simulink model "trans_canal_recep_2015a"  (R2015a)
settings: Solver=ode45  SolverMode=SingleTasking  StartTime=0.0  StopTime=100  MaxStep=0.001  RelTol=1e-3
InitFcn:
  | cd(tempdir)
  | clearvars
  | clc
  | 
  | %Carrossel?
  | mode_t=1;
  | 
  | %Depuração?
  | dep=0;
  | 
  | %Parâmetros do transmissor
  | fs_Tx=200e3;
  | f_bits=10e3;
  | rolloff=0.5;
  | smpl_per_symb=5;
  | [N,D]=rat(400000/(f_bits*smpl_per_symb));
  | rate_inter=(N);
  | rate_dec=(D);
  | 
  | %Canal
  | noise_pwr=0.25;
  | freq_canal=500;
  | att_canal=0.001;
  | 
  | 
  | %Barker e coef. do filtro casado
  | bark=[3 3 3 3 3 0 0 3 3 0 3 0 3 3 3 2 1 2 2 3 3 3 0 3 1 1];
  | y = pskmod(bark,4,pi/4,'gray');
  | coef=flip(conj(y));
  | 
  | 
  | %%%RECEPTOR%%%
  | 
  | Rsymbol = f_bits/2;                     % QPSK, so 2 samples per symbol
  | fs_Rx = 240e3;                            % sampling rate in the receiver
  | Rx_dec=6;
  | Rx_int=2;
  | OSR = (fs_Rx*Rx_int/(Rx_dec))/Rsymbol;     % oversampling ratio used in timing and frequency synch
  | smpl_per_symb_rec=fs_Rx/(Rx_dec*Rsymbol);
  | 
  | if f_bits==2e3
  |    nbw=0.00095;
  |    zeta=1.2;
  | else
  |    nbw=0.001;
  |    zeta=1.1;
  | end
  | 
  | %Largura de banda norm. do sinc. de portadora
  | if f_bits==40e3
  |     c_nbw=0.05;
  | else
  |     c_nbw=0.1;
  | end
  | 
  | %data='The man in black fled across the desert, and the gunslinger followed. The desert was the apotheosis of all deserts, huge, standing to the sky for what might have been parsecs in all directions. White; blinding; waterless; without feature save for the faint, cloudy haze of the mountains which sketched themselves on the horizon and the devil-grass which brought sweet dreams, nightmares, death. An occasional tombstone sign pointed the way, for once the drifted track that cut its way through the thick crust of alkali had been a highway and coaches had followed it. The world had moved on since then. The world had emptied. The gunslinger walked stolidly, not hurrying, not loafing. A hide waterbag was slung around his middle like a bloated sausage. It was almost full. He had progressed through the khef over many years, and had reached the fifth level. At the seventh or eighth, he would not have been thirsty; he could have watched own body dehydrate with clinical, detached attention, watering its crevices and dark inner hollows only when his logic told him it must be done. He was not seventh or eighth. He was fifth. So he was thirsty, although he had no particular urge to drink. In a vague way, all this pleased him. It was romantic. Below the waterbag were his guns, finely weighted to his hand. The two belts crisscrossed above his crotch. The holsters were oiled too deeply for even this Philistine sun to crack. The stocks of the guns were sandalwood, yellow and finely grained. The holsters were tied down with raw hide cord, and they swung heavily against his hips. The brass casings of the cartridges looped into the gun belts twinkled and flashed and heliographed in the sun. The leather made subtle creaking noises. The guns themselves made no noise. They had spilled blood. There was no need to make noise in the sterility of the desert His clothes were the no-color of rain or dust. His shirt was open at the throat, with a rawhide thong dangling loosely in hand-punched eyelets. His pants were seam-stretched dungarees. He breasted a gently rising dune (although there was no sand here; the desert was hardpan, and even the harsh winds that blew when dark came raised only an aggravating harsh dust like scouring powder) and saw the kicked remains of a tiny campfire on the lee side, the side which the sun would quit earliest. Small signs like this, once more affirming the man in black´s essential humanity, never failed to please him. His lips stretched in the pitted, flaked remains of his face. He squatted. He had burned the devil-grass, of course. It was the only thing out here that would burn. It burned with a greasy, flat light, and it burned slow. Border dwellers had told him that devils lived even in the flames. They burned it but would not look into the light. They said the devils hypnotized, beckoned, would eventually draw the one who looked into the fires. And the next man foolish enough to look into the fire might see you. The burned grass was crisscrossed in the now-familiar ideographic pattern, and crumbled to gray senselessness before the gunslinger´s prodding hand. There was nothing in the remains but a charred scrap of bacon, which he ate thoughtfully. It had always been this way. The gunslinger had followed the man in black across the desert for two months now, across the endless, screamingly monotonous purgatorial wastes, and had yet to find spoor other than the hygienic sterile ideographs of the man in black´s camp fires. He had not found a can, a bottle, or a waterbag (the gunslinger had left four of those behind, like dead snake-skins).';
  | data='The man in black fled across the desert, and the gunslinger followed. The desert was the apotheosis of all deserts, huge, standing to the sky for what might have been parsecs in all directions. White; blinding; waterless; without feature save for the faint, cloudy haze of the mountains which sketched themselves on the horizon and the devil-grass which brought sweet dreams, nightmares, death. An occasional tombstone sign pointed the way, for once the drifted track that cut its way through the thick crust of alkali had been a highway and coaches had followed it. The world had moved on since then.';
undefined symbols (not defined in the file): firnyquist, jsin
libraries: dspmlti4 x5, commdigbbndpm3 x3, dspsrcs4 x2, commfilt2 x2, commrfcorlib x1, simulink x1
settings Model: CovMetricSettings=dwe  CovHtmlReporting=off  covSaveCumulativeToWorkspaceVar=off  CovSaveSingleToWorkspaceVar=off  CovExternalEMLEnable=on  Creator=Enrique Pinto  LastModifiedBy=Enrique Pinto
settings DataIOCC: LimitDataPoints=off  SaveFormat=Dataset
settings DebuggingCC: SFUnexpectedBacktrackingDiag=error  SFNoUnconditionalDefaultTransitionDiag=error
settings HardwareCC: ProdBitPerPointer=64  ProdLargestAtomicFloat=Float  ProdIntDivRoundTo=Zero  ProdEndianess=LittleEndian  ProdHWDeviceType=Specified
settings ModelReferenceCC: PropagateSignalLabelsOutOfModel=on
settings GRTTargetCC: TargetLangStandard=C99 (ISO)  GeneratePreprocessorConditionals=Use local settings

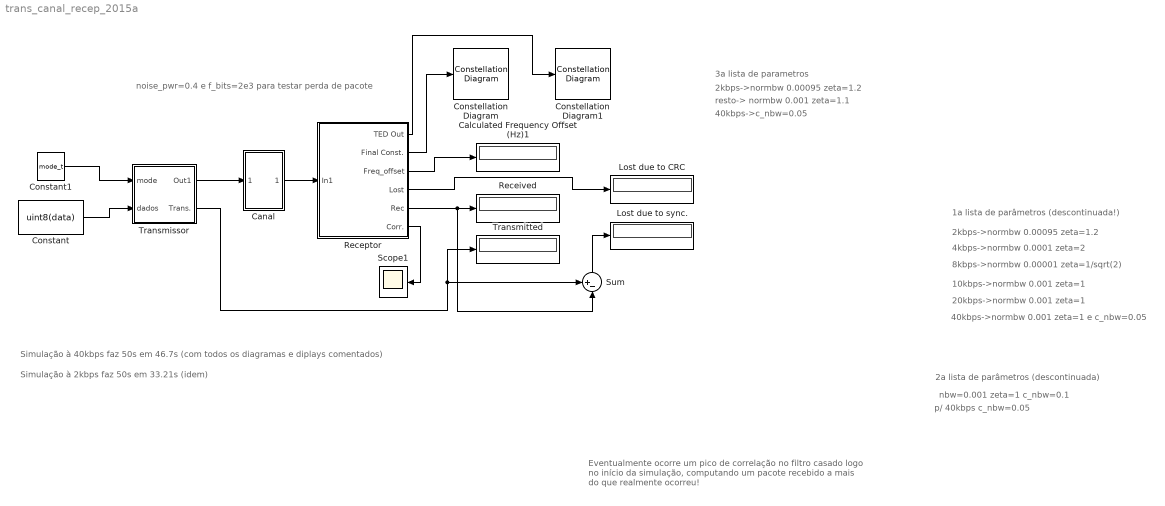
== system trans_canal_recep_2015a ==
  note: 40kbps->c_nbw=0.05
  note: resto-> normbw 0.001 zeta=1.1
  note: 2kbps->normbw 0.00095 zeta=1.2
  note: 3a lista de parametros
  note: Simulação à 2kbps faz 50s em 33.21s (idem)
  note: Simulação à 40kbps faz 50s em 46.7s (com todos os diagramas e diplays comentados)
  note: p/ 40kbps c_nbw=0.05
  note: nbw=0.001 zeta=1 c_nbw=0.1
  note: 2a lista de parâmetros (descontinuada)
  note: 1a lista de parâmetros (descontinuada!)
  note: Eventualmente ocorre um pico de correlação no filtro casado
      | logo no início da simulação, computando um pacote recebido
      | a mais do que realmente ocorreu!
  note: noise_pwr=0.4 e f_bits=2e3 para testar perda de pacote
  note: 10kbps->normbw 0.001 zeta=1
  note: 8kbps->normbw 0.00001 zeta=1/sqrt(2)
  note: 4kbps->normbw 0.0001 zeta=2
  note: 2kbps->normbw 0.00095 zeta=1.2
  note: 20kbps->normbw 0.001 zeta=1
  note: 40kbps->normbw 0.001 zeta=1 e c_nbw=0.05
  Calculated Frequency Offset (Hz)1 : Display
  Canal : Subsystem  mask{noise_pwr=noise_pwr, freq_channel=freq_canal}
      mask prompts: noise_pwr "Noise Power"; freq_channel "Frequency Deviation"
  Constant : Constant  Value=uint8(data)
  Constant1 : Constant  Value=mode_t
  Constellation Diagram : ConstellationDiagram
  Constellation Diagram1 : ConstellationDiagram
  Lost due to CRC : Display
  Lost due to sync. : Display
  Received : Display
  Receptor : Subsystem
  Scope1 : Scope
      settings: TimeRange=auto  MaxDataPoints=5000  SaveToWorkspace=off  SaveName=ScopeData  YMin=-6.73795  YMax=60.64159  SampleTime=-1
  Sum : Sum  Inputs=+-|
  Transmissor : Subsystem
  Transmitted : Display
  wires:
  Constant1/1 -> Transmissor/1(mode)
  Constant/1 -> Transmissor/2(dados)
  Receptor/1(TED Out) -> Constellation Diagram1/1
  Receptor/2(Final Const.) -> Constellation Diagram/1
  Receptor/3(Freq_offset) -> Calculated Frequency Offset (Hz)1/1
  Receptor/4("Lost ") -> Lost due to CRC/1
  Receptor/5("Rec ") -> Sum/2, Received/1
  Transmissor/2(Trans.) -> Transmitted/1, Sum/1
  Receptor/6("Corr. ") -> Scope1/1
  Sum/1 -> Lost due to sync./1
  Transmissor/1(Out1) -> Canal/1(In1)
  Canal/1(Out1) -> Receptor/1(In1)

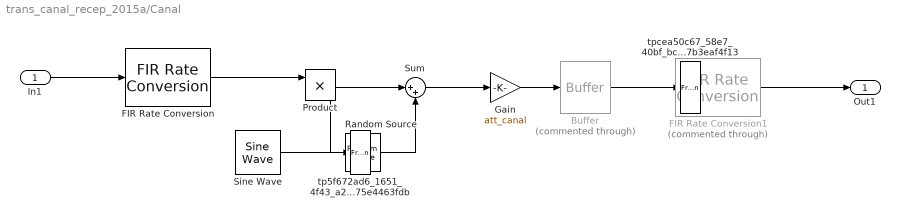
== system trans_canal_recep_2015a/Canal ==
  In1 : Inport
  Buffer : Buffer  Commented=through  N=10000
  FIR Rate Conversion : dspmlti4/FIR Rate Conversion  FilterSource=Specify via dialog  L=6  h=6 .* firnyquist(24*max(6,5), max(6,5), kaiser(1 + 24*max(6,5), 0.1102*(80-8.71)))  M=5  FilterObject=FRC  roundingMode=Floor  overflowMode=off  firstCoeffDataTypeStr=Inherit: Same word length as input  firstCoeffMin=[]  firstCoeffMax=[]  firstCoeffLastDataTypeStr=Inherit: Same word length as input  outputDataTypeStr=Inherit: Same as accumulator  outputMin=[]  outputMax=[]  outputLastDataTypeStr=Inherit: Same as accumulator
  FIR Rate Conversion1 : dspmlti4/FIR Rate Conversion  Commented=through  FilterSource=Specify via dialog  L=10060  h=10060 .* firnyquist(24*max(10060,10000), max(10060,10000), kaiser(1 + 24*max(10060,10000), 0.1102*(80-8.71)))  M=10000  FilterObject=FRC  roundingMode=Floor  overflowMode=off  firstCoeffDataTypeStr=Inherit: Same word length as input  firstCoeffMin=[]  firstCoeffMax=[]  firstCoeffLastDataTypeStr=Inherit: Same word length as input  outputDataTypeStr=Inherit: Same as accumulator  outputMin=[]  outputMax=[]  outputLastDataTypeStr=Inherit: Same as accumulator
  Gain : Gain  Gain=att_canal
  Product : Product
  Random Source : dspsrcs4/Random Source  SrcType=Gaussian  NormMethod=Ziggurat  CltLength=12  MinVal=0  MaxVal=1  MeanVal=0  VarVal=noise_pwr  RepMode=Not repeatable  rawSeed=1  IsInherit=off  SampMode=Discrete  SampTime=1/240000  SampFrame=1200  DataType=Double  OutComplex=Real
  Sine Wave : dspsrcs4/Sine Wave  Amplitude=1  Frequency=freq_channel  Phase=0  SampleMode=Discrete  OutComplex=Complex  CompMethod=Trigonometric fcn  TableSize=Speed  SampleTime=1/240000  SamplesPerFrame=1200  ResetState=Restart at time zero  dataType=double  wordLen=16  udDataType=sfix(16)  fracBitsMode=Best precision  numFracBits=15  OutDataTypeStr=double  LastOutDataTypeStr=double
  Sum : Sum  Inputs=|++
  tp5f672ad6_1651_4f43_a20c_0475e4463fdb : FrameConversion  InheritSamplingMode=off  OutFrame=Sample-based
  tpcea50c67_58e7_40bf_bc72_a47b3eaf4f13 : FrameConversion  InheritSamplingMode=off  OutFrame=Sample-based
  Out1 : Outport
  wires:
  Product/1 -> Sum/1
  Random Source/1 -> Sum/2
  Sum/1 -> Gain/1
  FIR Rate Conversion/1 -> Product/1
  Gain/1 -> Buffer/1
  In1/1 -> FIR Rate Conversion/1
  FIR Rate Conversion1/1 -> Out1/1
  Sine Wave/1 -> tp5f672ad6_1651_4f43_a20c_0475e4463fdb/1
  tp5f672ad6_1651_4f43_a20c_0475e4463fdb/1 -> Product/2
  Buffer/1 -> tpcea50c67_58e7_40bf_bc72_a47b3eaf4f13/1
  tpcea50c67_58e7_40bf_bc72_a47b3eaf4f13/1 -> FIR Rate Conversion1/1

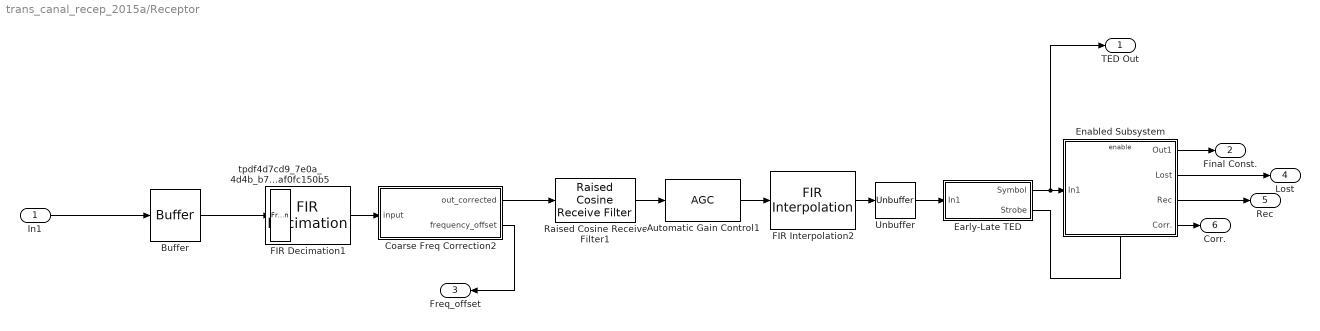
== system trans_canal_recep_2015a/Receptor ==
  In1 : Inport
  Automatic Gain Control1 : commrfcorlib/AGC  DetectorMethod=Rectifier  LoopMethod=Linear  UpdatePeriod=128  StepSize=0.05  MaximumGain=20  GainOutputPort=off  SimulateUsing=Code generation
  Buffer : Buffer  N=4096
  Coarse Freq Correction2 : Subsystem  mask{M=4, fs=fs_Rx/Rx_dec}
      mask prompts: M "Number of Symbols"; fs "Sample Frequency"
  Early-Late TED : Subsystem  mask{OSR=OSR, Bn=nbw, z=zeta}
      mask prompts: OSR "Oversampling Rate (OSR)"; Bn "Norm. BW"; z "Zeta"
      mask init:
      | % *** SYMBOL TIMING synch loop ***
      | Kp= 1;
      | Ko= 1;
      | n=(Bn)/(z+(1/(4*z)));
      | Ka=4*z*n/(Ko*Kp*(1+2*z*n+n^2));
      | Kb=4*(n^2)/(Ko*Kp*(1+2*z*n+n^2));
      mask DialogControl DescGroupVar Prompt: Early-Late TED
  Enabled Subsystem : Subsystem  TreatAsAtomicUnit=on
  FIR Decimation1 : dspmlti4/FIR Decimation  FilterSource=Specify via dialog  h=fir1(Rx_dec*10,1/Rx_dec)  D=Rx_dec  filtStruct=Direct form  FilterObject=Hm_firdecim  InputProcessing=Columns as channels (frame based)  framing=Allow multirate processing  inputOffset=0  outputBufInitCond=0  roundingMode=Floor  overflowMode=off  firstCoeffDataTypeStr=Inherit: Same word length as input  firstCoeffMin=[]  firstCoeffMax=[]  firstCoeffLastDataTypeStr=Inherit: Same word length as input  outputDataTypeStr=Inherit: Same as accumulator  outputMin=[]  outputMax=[]  outputLastDataTypeStr=Inherit: Same as accumulator
  FIR Interpolation2 : dspmlti4/FIR Interpolation  FilterSource=Specify via dialog  h=Rx_int*fir1(Rx_int*10,1/Rx_int)  L=Rx_int  FilterObject=Hm_firinterp  InputProcessing=Columns as channels (frame based)  framing=Enforce single-rate processing  outputBufInitCond=0  roundingMode=Floor  overflowMode=off  firstCoeffDataTypeStr=Inherit: Same word length as input  firstCoeffMin=[]  firstCoeffMax=[]  firstCoeffLastDataTypeStr=Inherit: Same word length as input  outputDataTypeStr=Inherit: Same as accumulator  outputMin=[]  outputMax=[]  outputLastDataTypeStr=Inherit: Same as accumulator
  Raised Cosine Receive Filter1 : commfilt2/Raised Cosine Receive Filter  filtType=Square root  R=rolloff  filtSpan=10  N=smpl_per_symb_rec  downFactor=1  downOffset=0  filterGain=1  InputProcessing=Columns as channels (frame based)  framing=Enforce single-rate processing  checkCoeff=off  variableName=rcRxFilt1  currentFiltSpan=10  D=(10)/2  sampMode=Mute  saveAsFlag=1  rateMode=Downsampling  checkGain=Normalized  launchFVT=on  roundingMode=Floor  overflowMode=off
  Unbuffer : Unbuffer  ic=0.7071+0.7071i
  tpdf4d7cd9_7e0a_4d4b_b754_45af0fc150b5 : FrameConversion  InheritSamplingMode=off  OutFrame=Sample-based
  TED Out : Outport
  Final Const. : Outport  Port=2
  Freq_offset : Outport  Port=3
  "Lost " : Outport  Port=4
  "Rec " : Outport  Port=5
  "Corr. " : Outport  Port=6
  wires:
  Coarse Freq Correction2/1(out_corrected) -> Raised Cosine Receive Filter1/1
  Unbuffer/1 -> Early-Late TED/1(In1)
  Automatic Gain Control1/1 -> FIR Interpolation2/1
  FIR Decimation1/1 -> Coarse Freq Correction2/1(input)
  Raised Cosine Receive Filter1/1 -> Automatic Gain Control1/1
  Early-Late TED/2(Strobe) -> Enabled Subsystem/Enable
  Early-Late TED/1(Symbol) -> TED Out/1, Enabled Subsystem/1(In1)
  FIR Interpolation2/1 -> Unbuffer/1
  Coarse Freq Correction2/2(frequency_offset) -> Freq_offset/1
  In1/1 -> Buffer/1
  Enabled Subsystem/1(Out1) -> Final Const./1
  Enabled Subsystem/2(Lost) -> "Lost "/1
  Enabled Subsystem/3("Rec ") -> "Rec "/1
  Enabled Subsystem/4(Corr.) -> "Corr. "/1
  Buffer/1 -> tpdf4d7cd9_7e0a_4d4b_b754_45af0fc150b5/1
  tpdf4d7cd9_7e0a_4d4b_b754_45af0fc150b5/1 -> FIR Decimation1/1

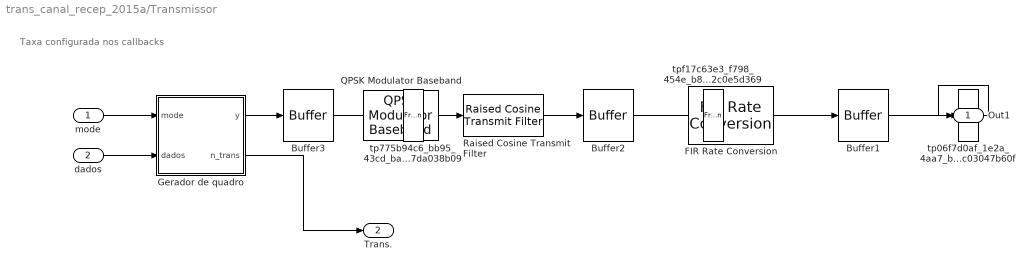
== system trans_canal_recep_2015a/Transmissor ==
  note: Taxa configurada nos callbacks
  mode : Inport
  dados : Inport  Port=2
  Buffer1 : Buffer  N=1000
  Buffer2 : Buffer  N=1000
  Buffer3 : Buffer  N=2
  FIR Rate Conversion : dspmlti4/FIR Rate Conversion  FilterSource=Specify via dialog  L=rate_inter  h=rate_inter .* firnyquist(24*max(rate_inter,rate_dec), max(rate_inter,rate_dec), kaiser(1 + 24*max(rate_inter,rate_dec), 0.1102*(80-8.71)))  M=rate_dec  FilterObject=FRC  roundingMode=Floor  overflowMode=off  firstCoeffDataTypeStr=Inherit: Same word length as input  firstCoeffMin=[]  firstCoeffMax=[]  firstCoeffLastDataTypeStr=Inherit: Same word length as input  outputDataTypeStr=Inherit: Same as accumulator  outputMin=[]  outputMax=[]  outputLastDataTypeStr=Inherit: Same as accumulator
  Gerador de quadro : MATLAB Function  TreatAsAtomicUnit=on  SystemSampleTime=1000/(f_bits)
      settings: PermitHierarchicalResolution=ParametersOnly
  QPSK Modulator Baseband : commdigbbndpm3/QPSK Modulator Baseband  InType=Bit  Enc=Gray  Ph=pi/4  outDtype=double  outWordLen=16  outUDDataType=sfix(16)  outFracLenMode=Best precision  outFracLen=15
  Raised Cosine Transmit Filter : commfilt2/Raised Cosine Transmit Filter  filtType=Square root  R=rolloff  filtSpan=10  N=smpl_per_symb  filterGain=1  InputProcessing=Columns as channels (frame based)  framing=Enforce single-rate processing  checkCoeff=off  variableName=rcTxFilt  checkGain=Normalized  sampMode=Mute  saveAsFlag=1  currentFiltSpan=10  D=(10)/2  launchFVT=on  roundingMode=Floor  overflowMode=off
  tp06f7d0af_1e2a_4aa7_b17e_2dc03047b60f : FrameConversion  InheritSamplingMode=off  OutFrame=Sample-based
  tp775b94c6_bb95_43cd_bac7_0de7da038b09 : FrameConversion  InheritSamplingMode=off  OutFrame=Sample-based
  tpf17c63e3_f798_454e_b87b_76c2c0e5d369 : FrameConversion  InheritSamplingMode=off  OutFrame=Sample-based
  Out1 : Outport
  Trans. : Outport  Port=2
  wires:
  FIR Rate Conversion/1 -> Buffer1/1
  Gerador de quadro/1(y) -> Buffer3/1
  mode/1 -> Gerador de quadro/1(mode)
  dados/1 -> Gerador de quadro/2(dados)
  QPSK Modulator Baseband/1 -> Raised Cosine Transmit Filter/1
  Gerador de quadro/2(n_trans) -> Trans./1
  Raised Cosine Transmit Filter/1 -> Buffer2/1
  Buffer1/1 -> tp06f7d0af_1e2a_4aa7_b17e_2dc03047b60f/1
  tp06f7d0af_1e2a_4aa7_b17e_2dc03047b60f/1 -> Out1/1
  Buffer2/1 -> tpf17c63e3_f798_454e_b87b_76c2c0e5d369/1
  tpf17c63e3_f798_454e_b87b_76c2c0e5d369/1 -> FIR Rate Conversion/1
  Buffer3/1 -> tp775b94c6_bb95_43cd_bac7_0de7da038b09/1
  tp775b94c6_bb95_43cd_bac7_0de7da038b09/1 -> QPSK Modulator Baseband/1

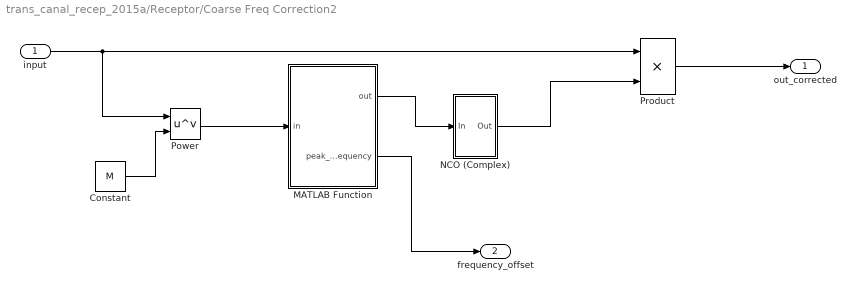
== system trans_canal_recep_2015a/Receptor/Coarse Freq Correction2 ==
  input : Inport
  Constant : Constant  Value=M  OutDataTypeStr=double
  MATLAB Function : MATLAB Function  TreatAsAtomicUnit=on
      settings: PermitHierarchicalResolution=ParametersOnly
  NCO (Complex) : Subsystem  mask{K=-2*pi/fs}
      mask prompts: K "Gain K"
  Power : Math  Operator=pow  OutputSignalType=complex  SaturateOnIntegerOverflow=on
  Product : Product
  out_corrected : Outport
  frequency_offset : Outport  Port=2
  wires:
  Power/1 -> MATLAB Function/1(in)
  Constant/1 -> Power/2
  MATLAB Function/1(out) -> NCO (Complex)/1(In)
  Product/1 -> out_corrected/1
  NCO (Complex)/1(Out) -> Product/2
  input/1 -> Power/1, Product/1
  MATLAB Function/2(peak_frequency) -> frequency_offset/1

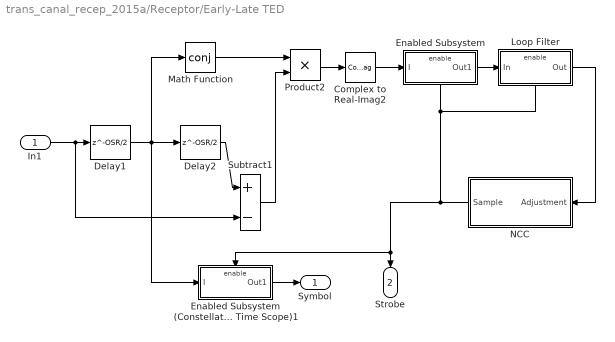
== system trans_canal_recep_2015a/Receptor/Early-Late TED ==
  In1 : Inport
  Complex to Real-Imag2 : ComplexToRealImag  Output=Real
  Delay1 : Delay  DelayLength=OSR/2
  Delay2 : Delay  DelayLength=OSR/2
  Enabled Subsystem : Subsystem  TreatAsAtomicUnit=on
  Enabled Subsystem (Constellation Diagram and Time Scope)1 : Subsystem  TreatAsAtomicUnit=on
  Loop Filter : Subsystem  TreatAsAtomicUnit=on
  Math Function : Math  Operator=conj  SaturateOnIntegerOverflow=on
  NCC : Subsystem  mask(Numerically Controller Clock (NCC)){OSR=OSR}
      mask prompts: OSR "Oversampling Ratio"
      mask help:
      | This component operates similarly to a Numerically Controlled Oscillator (NCO).
      |
      | Internally, a nominal step size of (1 + Adjustment) is applied to an accumulator. The accumulator wraps around at N = OSR, therefore for a zero control input, the accumulator wraps once every symbol period at the expected rate.
      |
      | When the accumulator wraps, a strobe output is produced.
  Product2 : Product
  Subtract1 : Sum  Inputs=+-
  Symbol : Outport
  Strobe : Outport  Port=2
  wires:
  Subtract1/1 -> Product2/2
  Delay2/1 -> Subtract1/1
  Complex to Real-Imag2/1 -> Enabled Subsystem/1(I)
  Enabled Subsystem (Constellation Diagram and Time Scope)1/1(Out1) -> Symbol/1
  Loop Filter/1(Out) -> NCC/1(Adjustment)
  Product2/1 -> Complex to Real-Imag2/1
  NCC/1(Sample) -> Enabled Subsystem (Constellation Diagram and Time Scope)1/Enable, Strobe/1, Loop Filter/Enable, Enabled Subsystem/Enable
  Delay1/1 -> Math Function/1, Delay2/1, Enabled Subsystem (Constellation Diagram and Time Scope)1/1(I)
  In1/1 -> Subtract1/2, Delay1/1
  Math Function/1 -> Product2/1
  Enabled Subsystem/1(Out1) -> Loop Filter/1(In)

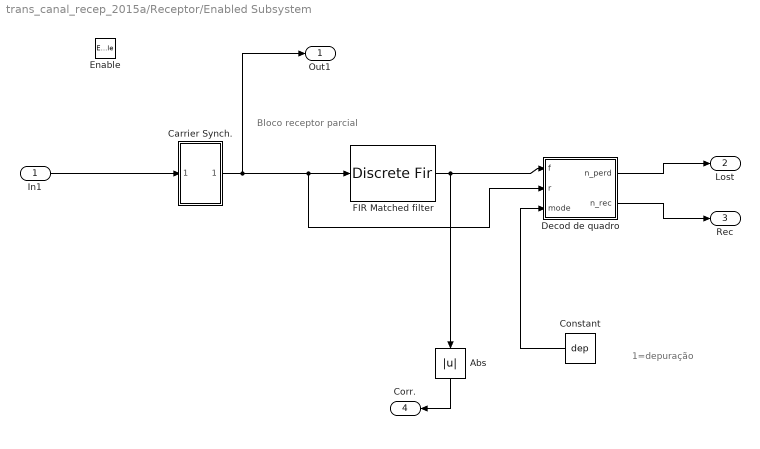
== system trans_canal_recep_2015a/Receptor/Enabled Subsystem ==
  note: 1=depuração
  note: Bloco receptor parcial
  In1 : Inport
  Enable : EnablePort
  Abs : Abs
  Carrier Synch. : Subsystem  mask(Carrier synch.){Bn=c_nbw}
      mask prompts: Bn "Normalized BW"
      mask init:
      | Kp= 0.5;
      | Ko= 1;
      | z= 1;
      | n=(Bn)/(z+(1/(4*z)));
      | K1=4*z*n/(Ko*Kp*(1+2*z*n+n^2));
      | K2=4*(n^2)/(Ko*Kp*(1+2*z*n+n^2));
  Constant : Constant  Value=dep
  "Decod de quadro " : MATLAB Function  TreatAsAtomicUnit=on
      settings: PermitHierarchicalResolution=ParametersOnly
  FIR Matched filter : DiscreteFir  Coefficients=coef
  Out1 : Outport
  Lost : Outport  Port=2
  "Rec " : Outport  Port=3
  Corr. : Outport  Port=4
  wires:
  In1/1 -> Carrier Synch./1(In1)
  Carrier Synch./1(Out1) -> Out1/1, "Decod de quadro "/2(r), FIR Matched filter/1
  Abs/1 -> Corr./1
  FIR Matched filter/1 -> "Decod de quadro "/1(f), Abs/1
  Constant/1 -> "Decod de quadro "/3(mode)
  "Decod de quadro "/1(n_perd) -> Lost/1
  "Decod de quadro "/2(n_rec) -> "Rec "/1

== system trans_canal_recep_2015a/Receptor/Coarse Freq Correction2/NCO (Complex) ==
  In : Inport
  Adder : DiscreteFilter  Denominator=[1 -1]  InputProcessing=Columns as channels (frame based)
  Gain : Gain  Gain=K
  Magnitude-Angle to Complex : MagnitudeAngleToComplex  Input=Angle  ConstantPart=1
  Out : Outport
  wires:
  In/1 -> Gain/1
  Magnitude-Angle to Complex/1 -> Out/1
  Gain/1 -> Adder/1
  Adder/1 -> Magnitude-Angle to Complex/1

== system trans_canal_recep_2015a/Receptor/Early-Late TED/Enabled Subsystem ==
  I : Inport
  Enable : EnablePort
  Out1 : Outport
  wires:
  I/1 -> Out1/1

== system trans_canal_recep_2015a/Receptor/Early-Late TED/Enabled Subsystem (Constellation Diagram and Time Scope)1 ==
  I : Inport
  Enable : EnablePort
  Out1 : Outport
  wires:
  I/1 -> Out1/1

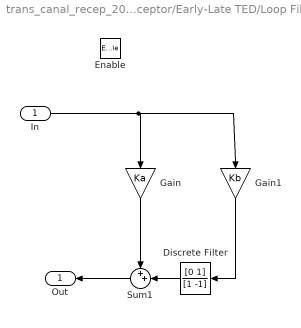
== system trans_canal_recep_2015a/Receptor/Early-Late TED/Loop Filter ==
  In : Inport
  Enable : EnablePort
  Discrete Filter : DiscreteFilter  Numerator=[0 1]  Denominator=[1 -1]  InputProcessing=Columns as channels (frame based)  FilterStructure=Direct form II transposed  a0EqualsOne=on
  Gain : Gain  Gain=Ka
  Gain1 : Gain  Gain=Kb
  Sum1 : Sum  Inputs=++|
  Out : Outport
  wires:
  Discrete Filter/1 -> Sum1/2
  Sum1/1 -> Out/1
  In/1 -> Gain1/1, Gain/1
  Gain1/1 -> Discrete Filter/1
  Gain/1 -> Sum1/1

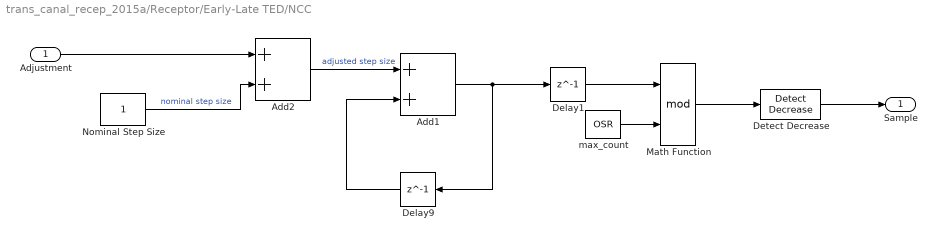
== system trans_canal_recep_2015a/Receptor/Early-Late TED/NCC ==
  Adjustment : Inport
  Add1 : Sum  OutDataTypeStr=double
  Add2 : Sum  OutDataTypeStr=double
  Delay1 : Delay  DelayLength=1
  Delay9 : Delay  DelayLength=1
  Detect Decrease : simulink/Logic and Bit Operations/Detect Decrease  vinit=0.0  InputProcessing=Inherited  OutDataTypeStr=boolean
  Math Function : Math  Operator=mod  SaturateOnIntegerOverflow=on
  Nominal Step Size : Constant  OutDataTypeStr=double  SampleTime=-1
  max_count : Constant  Value=OSR  OutDataTypeStr=double  SampleTime=-1
  Sample : Outport
  wires:
  Adjustment/1 -> Add2/1
  Add2/1 -> Add1/1  "adjusted step size"
  Delay9/1 -> Add1/2
  Nominal Step Size/1 -> Add2/2  "nominal step size"
  Add1/1 -> Delay9/1, Delay1/1
  Math Function/1 -> Detect Decrease/1
  max_count/1 -> Math Function/2
  Detect Decrease/1 -> Sample/1
  Delay1/1 -> Math Function/1

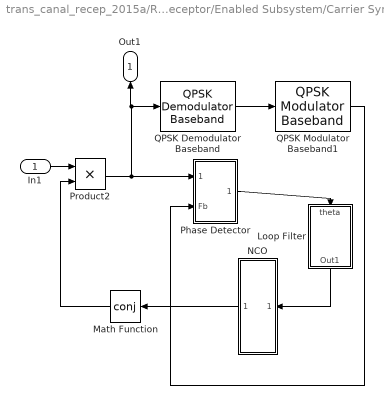
== system trans_canal_recep_2015a/Receptor/Enabled Subsystem/Carrier Synch. ==
  In1 : Inport
  Loop Filter : Subsystem
  Math Function : Math  Operator=conj  SaturateOnIntegerOverflow=on
  NCO : Subsystem
  Phase Detector : Subsystem
  Product2 : Product
  QPSK Demodulator Baseband : commdigbbndpm3/QPSK Demodulator Baseband  OutType=Integer  DecType=Hard decision  VarSource=Dialog  Variance=1  Dec=Gray  Ph=pi/4  outDtype1=Inherit via internal rule  outDtype2=Inherit via internal rule  derotateFactorWordLen=16
  QPSK Modulator Baseband1 : commdigbbndpm3/QPSK Modulator Baseband  InType=Integer  Enc=Gray  Ph=pi/4  outDtype=double  outWordLen=16  outUDDataType=sfix(16)  outFracLenMode=Best precision  outFracLen=15
  Out1 : Outport
  wires:
  Phase Detector/1(Out1) -> Loop Filter/1(theta)
  QPSK Demodulator Baseband/1 -> QPSK Modulator Baseband1/1
  NCO/1(z[n]) -> Math Function/1
  Math Function/1 -> Product2/2
  Product2/1 -> QPSK Demodulator Baseband/1, Out1/1, Phase Detector/1(Ref)
  QPSK Modulator Baseband1/1 -> Phase Detector/2(Fb)
  Loop Filter/1(Out1) -> NCO/1(v[m])
  In1/1 -> Product2/1

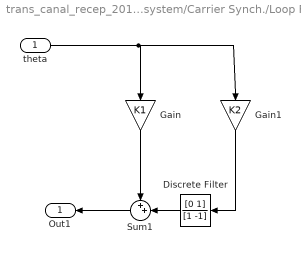
== system trans_canal_recep_2015a/Receptor/Enabled Subsystem/Carrier Synch./Loop Filter ==
  theta : Inport
  Discrete Filter : DiscreteFilter  Numerator=[0 1]  Denominator=[1 -1]  InputProcessing=Columns as channels (frame based)  FilterStructure=Direct form II transposed  a0EqualsOne=on
  Gain : Gain  Gain=K1
  Gain1 : Gain  Gain=K2
  Sum1 : Sum  Inputs=++|
  Out1 : Outport
  wires:
  Gain/1 -> Sum1/1
  Gain1/1 -> Discrete Filter/1
  theta/1 -> Gain1/1, Gain/1
  Sum1/1 -> Out1/1
  Discrete Filter/1 -> Sum1/2

== system trans_canal_recep_2015a/Receptor/Enabled Subsystem/Carrier Synch./NCO ==
  v[m] : Inport
  Delay : Delay  DelayLength=1  InitialCondition=0  InputProcessing=Columns as channels (frame based)
  Sum1 : Sum  Inputs=++|
  Trigonometric Function : Trigonometry  Operator=cos + jsin
  z[n] : Outport
  wires:
  v[m]/1 -> Sum1/2
  Sum1/1 -> Delay/1
  Trigonometric Function/1 -> z[n]/1
  Delay/1 -> Sum1/1, Trigonometric Function/1

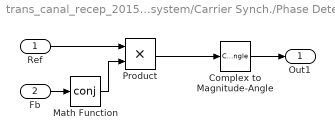
== system trans_canal_recep_2015a/Receptor/Enabled Subsystem/Carrier Synch./Phase Detector ==
  Ref : Inport
  Fb : Inport  Port=2
  Complex to Magnitude-Angle : ComplexToMagnitudeAngle  Output=Angle
  Math Function : Math  Operator=conj  SaturateOnIntegerOverflow=on
  Product : Product
  Out1 : Outport
  wires:
  Product/1 -> Complex to Magnitude-Angle/1
  Math Function/1 -> Product/2
  Complex to Magnitude-Angle/1 -> Out1/1
  Fb/1 -> Math Function/1
  Ref/1 -> Product/1

== matlab function trans_canal_recep_2015a/Transmissor/Gerador de quadro ==
  data: mode input; y output; dados input; n_trans output
function [y,n_trans] = fcn(mode,dados)
persistent databuf;
if isempty(databuf)
    %A opção abaixo funciona
    %databuf=uint8('The man in black fled across the desert, and the gunslinger followed. The desert was the apotheosis of all deserts, huge, standing to the sky for what might have been parsecs in all directions. White; blinding; waterless; without feature save for the faint, cloudy haze of the mountains which sketched themselves on the horizon and the devil-grass which brought sweet dreams, nightmares, death. An occasional tombstone sign pointed the way, for once the drifted track that cut its way through the thick crust of alkali had been a highway and coaches had followed it. The world had moved on since then. The world had emptied. The gunslinger walked stolidly, not hurrying, not loafing. A hide waterbag was slung around his middle like a bloated sausage. It was almost full. He had progressed through the khef over many years, and had reached the fifth level. At the seventh or eighth, he would not have been thirsty; he could have watched own body dehydrate with clinical, detached attention, watering its crevices and dark inner hollows only when his logic told him it must be done. He was not seventh or eighth. He was fifth. So he was thirsty, although he had no particular urge to drink. In a vague way, all this pleased him. It was romantic. Below the waterbag were his guns, finely weighted to his hand. The two belts crisscrossed above his crotch. The holsters were oiled too deeply for even this Philistine sun to crack. The stocks of the guns were sandalwood, yellow and finely grained. The holsters were tied down with raw hide cord, and they swung heavily against his hips. The brass casings of the cartridges looped into the gun belts twinkled and flashed and heliographed in the sun. The leather made subtle creaking noises. The guns themselves made no noise. They had spilled blood. There was no need to make noise in the sterility of the desert His clothes were the no-color of rain or dust. His shirt was open at the throat, with a rawhide thong dangling loosely in hand-punched eyelets. His pants were seam-stretched dungarees. He breasted a gently rising dune (although there was no sand here; the desert was hardpan, and even the harsh winds that blew when dark came raised only an aggravating harsh dust like scouring powder) and saw the kicked remains of a tiny campfire on the lee side, the side which the sun would quit earliest. Small signs like this, once more affirming the man in black´s essential humanity, never failed to please him. His lips stretched in the pitted, flaked remains of his face. He squatted. He had burned the devil-grass, of course. It was the only thing out here that would burn. It burned with a greasy, flat light, and it burned slow. Border dwellers had told him that devils lived even in the flames. They burned it but would not look into the light. They said the devils hypnotized, beckoned, would eventually draw the one who looked into the fires. And the next man foolish enough to look into the fire might see you. The burned grass was crisscrossed in the now-familiar ideographic pattern, and crumbled to gray senselessness before the gunslinger´s prodding hand. There was nothing in the remains but a charred scrap of bacon, which he ate thoughtfully. It had always been this way. The gunslinger had followed the man in black across the desert for two months now, across the endless, screamingly monotonous purgatorial wastes, and had yet to find spoor other than the hygienic sterile ideographs of the man in black´s camp fires. He had not found a can, a bottle, or a waterbag (the gunslinger had left four of those behind, like dead snake-skins).$$$$$$$$$$$$$$$$$$$$$$$$$$$$$$$$');
    %A opção abaixo carrega no buffer apenas o primeiro elemento de dados!
    databuf=uint8(zeros(1,length(dados)));
    databuf(1:length(dados))=dados(1:length(dados));
end
persistent i;
if isempty(i)
    i=1;
end
persistent n_count;
if isempty(n_count)
    n_count=0;
end
frame=zeros(1,984);
%Barker 13 =>[1 1 1 1 1 0 0 1 1 0 1 0 1]
%Preâmbulo de sincronismo
frame(1:52)=[1 1 1 1 1 1 1 1 1 1 0 0 0 0 1 1 1 1 0 0 1 1 0 0 1 1 1 1 1 1 1 0 0 1 1 0 1 0 1 1 1 1 1 1 0 0 1 1 0 1 0 1];
%Modo
frame(53:55)=zeros(1,3);
frame(56)=mode;

%Índice
frame(57:64-size(de2bi(i-1),2))=zeros(1,8-size(de2bi(i-1),2));
frame(64-size(de2bi(i-1),2)+1:64)=fliplr(de2bi(i-1));

%End_flag e carrossel
texto=uint8('vazio');
texto=texto';

databuf=uint8(zeros(1,length(dados)));
databuf(1:length(dados))=dados(1:length(dados));
    
if(mode==1)%verifica se é carrossel
    carrossel_size=ceil(size(databuf,2)/114);
    if(i==carrossel_size)
        frame(65)=1;
        texto=databuf((i-1)*114+1:(size(databuf,2)));
        i=1;
    else
        if(i<carrossel_size)
            texto=databuf((i-1)*114+1:i*114);
            i=i+1;
        else
            i=1;
        end
    end
else
    texto=databuf(1:114);
    texto=texto.';
    if(i==256)
        frame(65)=1;
        i=1;
    else
        if(i<256)
            i=i+1;
        else
            i=1;
        end
    end
end

%Tamanho mensagem
frame(66:72-size(dec2bin(size(dec2bin(texto),1)),2))=zeros(1,7-size(dec2bin(size(dec2bin(texto),1)),2));
frame(72-size(dec2bin(size(dec2bin(texto),1)),2)+1:72)=dec2bin(size(dec2bin(texto),1));
%Dados
mensagem = reshape(dec2bin(texto, 8).'-'0',1,[]);
frame(73:73+size(mensagem,2)-1)=mensagem';
frame(73+size(mensagem,2):984)=randi([0 1],1,984-(73+size(mensagem,2))+1);
%Output
H = comm.CRCGenerator;
y_sem_pre=step(H,frame(53:end)');
y=[frame(1:52)'; y_sem_pre];
n_count=n_count+1;
n_trans=n_count;

== matlab function trans_canal_recep_2015a/Receptor/Coarse Freq Correction2/MATLAB Function ==
  data: in input; out output; fs parameter; M parameter; peak_frequency output
function [out, peak_frequency]= fcn(in, fs, M)
length_signal = size(in, 1);
fft_signal = abs(fftshift(fft(in, length_signal)));
frequencies = linspace(-fs/2, fs/2, length_signal);
[value, peak_index] = max(fft_signal);
peak_frequency = frequencies(peak_index)/M;
out_vector = ones(length_signal, 1);
out = peak_frequency * out_vector;

== matlab function trans_canal_recep_2015a/Receptor/Enabled Subsystem/Decod de quadro  ==
  data: f input; r input double; mode input; n_perd output; n_rec output
function [n_perd,n_rec]=fcn(f,r,mode)
coder.extrinsic('num2str')
coder.extrinsic('cprintf')
G = comm.CRCDetector;
H = comm.QPSKDemodulator('PhaseOffset',pi/4,'BitOutput',true);
persistent mode_r;
if isempty(mode_r)
    mode_r=1;
end
persistent rec_count;
if isempty(rec_count)
    rec_count=0;
end
persistent lost_count;
if isempty(lost_count)
    lost_count=0;
end

persistent flag_size;
if isempty(flag_size)
    flag_size=0;
end
persistent indices_rec;
if isempty(indices_rec)
    indices_rec=zeros(256,1);
end
persistent index_max;
if isempty(index_max)
    index_max=0;
end
persistent msg_buf;
if isempty(msg_buf)
    msg_buf=char(zeros(29184,1)); %114*256 de tamanho
end
persistent msg_qpsk;
if isempty(msg_qpsk)
    msg_qpsk=complex(zeros(500-26,1));
end
persistent f_angle;
if isempty(f_angle)
    f_angle=0;
end
persistent enable;
if isempty(enable)
    enable = 0;
end
persistent k;
if isempty(k)
    k = 0;
end

if (abs(f)>22)&&(enable==0)
    enable=1;
    k=0;
    f_angle=angle(f);
    rec_count=rec_count+1;
end

if enable==1
    if (k<(500-26+1))
        if(k>0)
            msg_qpsk(k)=r;
        end
        k=k+1;
    else
        enable=0;
        msg = H(exp(-1i*f_angle)*msg_qpsk);
        [~,err] = G(msg);
        if err==1
            lost_count=lost_count+1;
        end
        if mode==0 %Se não for depuração...
            % Comentado abaixo está o programa de teste
%                                     mode_r=char(msg(56-52)+48);
%                                     index=num2str(bi2de(reshape(msg(57-52:64-52),8,[])','left-msb')');
%                                     endflag = msg(65-52);
%                                     datasize= num2str(bi2de(reshape(msg(66-52:72-52),7,[])','left-msb')');
%                                     data = char(bi2de(reshape(msg(73-52:984-52),8,[])','left-msb')');
%                                     fwrite(fid,data);
%                                     fprintf(fid,'\n');
%                                     fprintf(2,'CRC:%d ',int8(err))
%                                     fprintf(2,'Index:%s ',index)
%                                     fprintf(2,'Flag:%d ',int8(endflag))
%                                     fprintf(2,'Size:%s ',datasize)
%                                     fprintf(2,'Msg:%s',data)
            if err==0 %Aguarda pacote sem erro para determinar o modo de transmissão

                mode_r=bi2de(msg(56-52));
                
                if mode_r==1 %Se carrossel... (Carrossel só processa pacotes sem erro!)
                    index=bi2de(reshape(msg(57-52:64-52),8,[])','left-msb')';
                    endflag = msg(65-52);
                    msg_buf((114*index+1):114*(index+1)) = char(bi2de(reshape(msg(73-52:984-52),8,[])','left-msb')');
                    indices_rec(index+1)=index+1;
                    if endflag==1
                        index_max=index+1;
                        flag_size=1;
                    else
                        index_max=max(indices_rec);
                    end
                    if(all(indices_rec(1:index_max))==1)&&(flag_size==1) %Verifica se recebeu todos os frames até o end flag
                        fprintf(2,'%s',msg_buf(1:index_max*114))
                        indices_rec=zeros(256,1);
                        index_max=0;
                        flag_size=0;
                        msg_buf=char(zeros(29184,1));
                    else %Caso não tenha redebido tudo, mostra o que recebeu
                        for i=1:index_max
                            if indices_rec(i)==0
                                fprintf(2,'-')
                            else
                                if (i==index_max)&&(flag_size==1)
                                    fprintf(2,'!') %Caso o caractere de maior índice seja com certeza o último, imprimir '!' em vez de '*'
                                else
                                    fprintf(2,'*')
                                end
                            end
                        end
                        fprintf(2,'/')%Imprime divisória entre quadros no display
                    end
                end
            end
            if mode_r==0 %Se contínuo...
                if err==1
                    fprintf(2,'___?___')
                else
                    data = char(bi2de(reshape(msg(73-52:984-52),8,[])','left-msb')');
                    fprintf(2,'%s',data)
                end
            end
            
            
            
            k=0;
        else %Se for depuração...
            if err==0
                index=num2str(bi2de(reshape(msg(57-52:64-52),8,[])','left-msb')');
                fprintf(2,'Rec:%s ',index)
            else
                fprintf(2,'error')
            end
        end
        
    end
end
n_perd=lost_count;
n_rec=rec_count;
